simulink model "model_harmonic2"  (Simulink 7.0)
settings: Solver=ode45  StartTime=0.0  StopTime=10.0  MaxStep=0.1  RelTol=1e-3
settings Model: Creator=peter  LastModifiedBy=peter  ExtModeAutoUpdateStatusClock=off

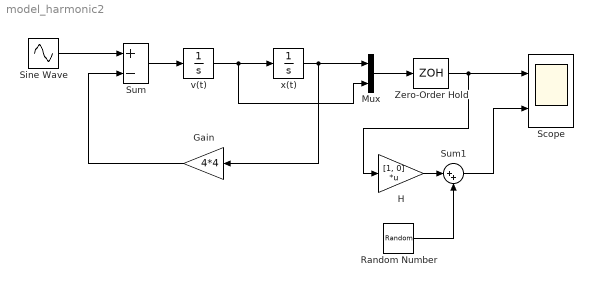
== system model_harmonic2 ==
  Gain : Gain  Orientation=left  Gain=4*4  ParameterDataType=sfix(16)  ParameterScaling=2^0  OutDataType=sfix(16)  OutScaling=2^0
  H : Gain  Gain=[1, 0]  Multiplication=Matrix(K*u)  ParameterDataType=sfix(16)  ParameterScaling=2^0  OutDataType=sfix(16)  OutScaling=2^0
  Mux : Mux  Inputs=2
  Random Number : RandomNumber  Variance=2e-4  SampleTime=0.05  VectorParams1D=off
  Scope : Scope  NumInputPorts=2
      settings: TimeRange=10  YMin=-1.1~-1.1  YMax=1.1~1.1
  Sine Wave : Sin  Frequency=3  SampleTime=0
  Sum : Sum  Inputs=+-  OutDataType=sfix(16)  OutScaling=2^0
  Sum1 : Sum  Inputs=|++  OutDataType=sfix(16)  OutScaling=2^0
  Zero-Order Hold : ZeroOrderHold  SampleTime=0.05
  v(t) : Integrator
  x(t) : Integrator
  wires:
  v(t)/1 -> x(t)/1, Mux/2
  x(t)/1 -> Gain/1, Mux/1
  Sum/1 -> v(t)/1
  Gain/1 -> Sum/2
  Sine Wave/1 -> Sum/1
  Mux/1 -> Zero-Order Hold/1
  Zero-Order Hold/1 -> H/1, Scope/1
  H/1 -> Sum1/1
  Random Number/1 -> Sum1/2
  Sum1/1 -> Scope/2
